simulink model "microgrid_healthy_load_profiling_with_Utility"  (Simulink 7.9)
settings: Solver=ode3  SolverMode=SingleTasking  StartTime=0.0  StopTime=12  FixedStep=1*10^(-4)  RelTol=1e-3
undefined symbols (not defined in the file): D1, Delta, Ts
libraries: powerlib x102, powerlib_extras x22
(part 1 of 2)
settings Model: Creator=SK  LastModifiedBy=SK
settings SolverCC: ZeroCrossAlgorithm=Adaptive  AlgebraicLoopSolver=LineSearch
settings OptimizationCC: SimCompilerOptimization=On  AccelVerboseBuild=on
settings SFSimCC: SFSimEnableDebug=off  SFSimEcho=off
settings RTWCC: RTWCompilerOptimization=On

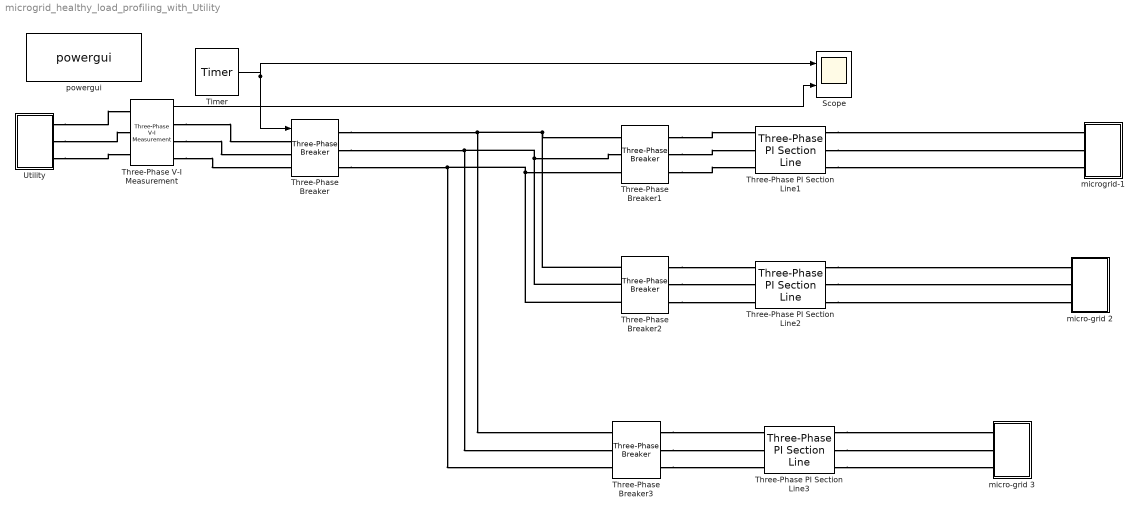
== system microgrid_healthy_load_profiling_with_Utility ==
  Scope : Scope  NumInputPorts=2
      settings: YMin=1~-55  YMax=1~55
  Three-Phase PI Section Line1 : powerlib/Elements/Three-Phase PI Section Line  LConnTagsString=a|b|c  RConnTagsString=A|B|C  Frequency=60  Resistances=[ 36.757 0.0]  Inductances="[ 0.126  0.0001]"  Capacitances=[0.00001 0.0001]  Length=2.06
  Three-Phase PI Section Line2 : powerlib/Elements/Three-Phase PI Section Line  LConnTagsString=a|b|c  RConnTagsString=A|B|C  Frequency=60  Resistances=[ 36.757 0.0]  Inductances="[ 0.126  0.0001]"  Capacitances=[0.00001 0.0001]  Length=2.06
  Three-Phase PI Section Line3 : powerlib/Elements/Three-Phase PI Section Line  LConnTagsString=a|b|c  RConnTagsString=A|B|C  Frequency=60  Resistances=[ 36.757 0.0]  Inductances="[ 0.126  0.0001]"  Capacitances=[0.00001 0.0001]  Length=2.06
  Three-Phase V-I Measurement : powerlib/Measurements/Three-Phase V-I Measurement  VoltageMeasurement=no  SetLabelV=off  LabelV=Vabc  Vpu=off  VpuLL=off  CurrentMeasurement=yes  SetLabelI=off  LabelI=Iabc  Ipu=off  Pbase=100e6  Vbase=500e3  OutputType=Magnitude  PhasorSimulation=off  PSBequivalent=0
  Three-Phase Breaker : powerlib/Elements/Three-Phase Breaker  InitialState=closed  SwitchA=on  SwitchB=on  SwitchC=on  SwitchTimes="[4/60  10/60]"  External=on  BreakerResistance=0.001  SnubberResistance=1e6  SnubberCapacitance=inf  Measurements=None
  Three-Phase Breaker1 : powerlib/Elements/Three-Phase Breaker  InitialState=open  SwitchA=off  SwitchB=off  SwitchC=off  SwitchTimes="[4/60  10/60]"  External=off  BreakerResistance=0.001  SnubberResistance=1e6  SnubberCapacitance=inf  Measurements=None
  Three-Phase Breaker2 : powerlib/Elements/Three-Phase Breaker  InitialState=open  SwitchA=off  SwitchB=off  SwitchC=off  SwitchTimes="[4/60  10/60]"  External=off  BreakerResistance=0.001  SnubberResistance=1e6  SnubberCapacitance=inf  Measurements=None
  Three-Phase Breaker3 : powerlib/Elements/Three-Phase Breaker  InitialState=open  SwitchA=off  SwitchB=off  SwitchC=off  SwitchTimes="[4/60  10/60]"  External=off  BreakerResistance=0.001  SnubberResistance=1e6  SnubberCapacitance=inf  Measurements=None
  Timer : powerlib_extras/Control  Blocks/Timer  t=[ 0 ]  e=[1]
  Utility : Subsystem
  micro-grid 2 : Subsystem
  micro-grid 3 : Subsystem
  microgrid-1 : Subsystem
  powergui : powerlib/powergui  Priority=1  SimulationMode=Discrete  SolverType=Tustin  SampleTime=Ts  frequency=60  SPID=on  DisableSnubberDevices=off  DisableRonSwitches=off  DisableVfSwitches=off  SwTol=0  Interpol=off  DisplayEquations=off  FunctionMessages=off  frequencyindice=60  Pbase=5e6  ErrMax=1e-4  Iterations=50  UnitsV=kV  UnitsW=MW  echomessages=off  HookPort=off  EnableUseOfTLC=off  x0status=blocks  RestoreLinks=warning  ResistiveCurrentMeasurement=off  Ylog=off  Xlog=on  ShowGrid=off  save=off  variable=ZData  structure=y  ZoomFFT=off  StartTime=0.0  cycles=1  DisplayStyle=1  fundamental=60  FreqAxis=off  MaxFrequency=1000  frequencyindicesteady=1  display=off  methode=off
  wires:
  Timer/1 -> Three-Phase Breaker/1, Scope/1
  Three-Phase V-I Measurement/1 -> Scope/2
  connections:
  Three-Phase V-I Measurement/RConn2 -- Three-Phase Breaker/LConn2
  Utility/RConn2 -- Three-Phase V-I Measurement/LConn2
  Three-Phase V-I Measurement/RConn1 -- Three-Phase Breaker/LConn1
  Three-Phase V-I Measurement/RConn3 -- Three-Phase Breaker/LConn3
  Utility/RConn1 -- Three-Phase V-I Measurement/LConn1
  Utility/RConn3 -- Three-Phase V-I Measurement/LConn3
  Three-Phase Breaker2/LConn1 -- Three-Phase Breaker/RConn1 -- Three-Phase Breaker3/LConn1 -- Three-Phase Breaker1/LConn1
  Three-Phase Breaker2/LConn2 -- Three-Phase Breaker/RConn2 -- Three-Phase Breaker3/LConn2 -- Three-Phase Breaker1/LConn2
  Three-Phase Breaker2/LConn3 -- Three-Phase Breaker/RConn3 -- Three-Phase Breaker3/LConn3 -- Three-Phase Breaker1/LConn3
  Three-Phase PI Section Line3/RConn1 -- micro-grid 3/LConn1
  Three-Phase PI Section Line3/RConn2 -- micro-grid 3/LConn2
  Three-Phase PI Section Line3/RConn3 -- micro-grid 3/LConn3
  Three-Phase PI Section Line1/RConn1 -- microgrid-1/LConn1
  Three-Phase PI Section Line1/RConn2 -- microgrid-1/LConn2
  Three-Phase PI Section Line1/RConn3 -- microgrid-1/LConn3
  Three-Phase PI Section Line2/RConn1 -- micro-grid 2/LConn1
  Three-Phase PI Section Line2/RConn2 -- micro-grid 2/LConn2
  Three-Phase PI Section Line2/RConn3 -- micro-grid 2/LConn3
  Three-Phase Breaker3/RConn1 -- Three-Phase PI Section Line3/LConn1
  Three-Phase Breaker3/RConn2 -- Three-Phase PI Section Line3/LConn2
  Three-Phase Breaker3/RConn3 -- Three-Phase PI Section Line3/LConn3
  Three-Phase Breaker2/RConn1 -- Three-Phase PI Section Line2/LConn1
  Three-Phase Breaker2/RConn2 -- Three-Phase PI Section Line2/LConn2
  Three-Phase Breaker2/RConn3 -- Three-Phase PI Section Line2/LConn3
  Three-Phase Breaker1/RConn1 -- Three-Phase PI Section Line1/LConn1
  Three-Phase Breaker1/RConn2 -- Three-Phase PI Section Line1/LConn2
  Three-Phase Breaker1/RConn3 -- Three-Phase PI Section Line1/LConn3

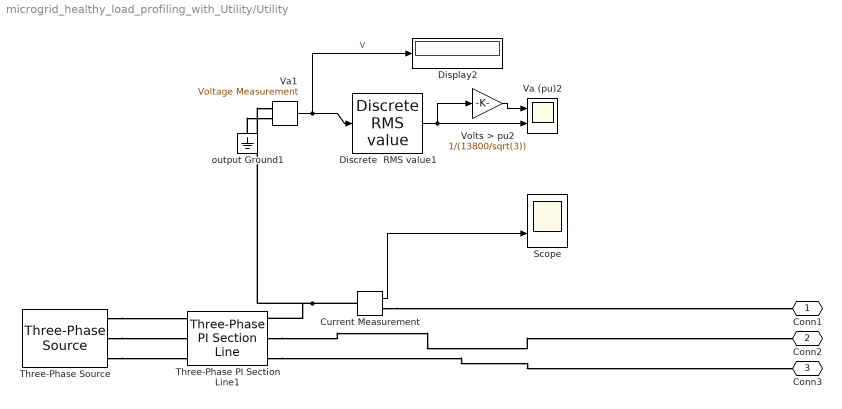
== system microgrid_healthy_load_profiling_with_Utility/Utility ==
  Current Measurement : powerlib/Measurements/Current Measurement  PhasorSimulation=off  OutputType=Complex  PSBequivalent=0
  Discrete  RMS value1 : powerlib_extras/Discrete Measurements/Discrete  RMS value  Freq=60  Mag_Init=0  Ts=Ts
  Display2 : Display
  Scope : Scope  NumInputPorts=2
      settings: YMin=-17500~-55  YMax=17500~55  SaveName=ScopeData2
  Three-Phase PI Section Line1 : powerlib/Elements/Three-Phase PI Section Line  LConnTagsString=a|b|c  RConnTagsString=A|B|C  Frequency=60  Resistances=[ 36.757 0.0]  Inductances="[ 0.126  0.0001]"  Capacitances=[0.00001 0.0001]  Length=2.06
  Three-Phase Source : powerlib/Electrical Sources/Three-Phase Source  Voltage=13.8e3  PhaseAngle=0  Frequency=60  InternalConnection=Yg  SpecifyImpedance=on  Resistance=0.8929  Inductance=16.58e-3  ShortCircuitLevel=1000e6  BaseVoltage=13.8e3  XRratio=22.2  BusType=swing  Pref=0  Qref=0  Qmin=-inf  Qmax=inf
  Va (pu)2 : Scope  NumInputPorts=2
      settings: TickLabels=on  TimeRange=3  YMin=1.35675~10809.8  YMax=1.35675~10809.8  SaveName=vf1
  Va1 : powerlib/Measurements/Voltage Measurement  Tag=PoWeRsYsTeMmEaSuReMeNt  PhasorSimulation=off  OutputType=Magnitude  PSBequivalent=0
  Volts > pu2 : Gain  Gain=1/(13800/sqrt(3))  SaturateOnIntegerOverflow=on  OutDataTypeStr=Inherit: Same as input  ParamDataTypeStr=Inherit: Same as input
  output Ground1 : powerlib/Elements/Ground  LConnTagsString=a
  Conn1 : PMIOPort  Port=1  Side=Right
  Conn2 : PMIOPort  Port=2  Side=Right
  Conn3 : PMIOPort  Port=3  Side=Right
  wires:
  Current Measurement/1 -> Scope/2
  Va1/1 -> Discrete  RMS value1/1, Display2/1  "V"
  Discrete  RMS value1/1 -> Va (pu)2/2, Volts > pu2/1
  Volts > pu2/1 -> Va (pu)2/1
  connections:
  Three-Phase Source/RConn1 -- Three-Phase PI Section Line1/LConn1
  Three-Phase Source/RConn2 -- Three-Phase PI Section Line1/LConn2
  Three-Phase Source/RConn3 -- Three-Phase PI Section Line1/LConn3
  Three-Phase PI Section Line1/RConn2 -- Conn2/RConn1
  Three-Phase PI Section Line1/RConn3 -- Conn3/RConn1
  Current Measurement/LConn1 -- Three-Phase PI Section Line1/RConn1 -- Va1/LConn1
  Current Measurement/RConn1 -- Conn1/RConn1
  output Ground1/LConn1 -- Va1/LConn2

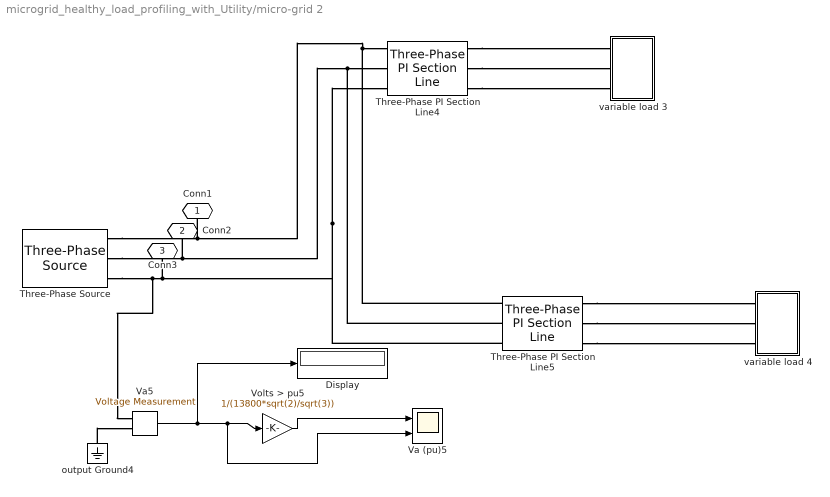
== system microgrid_healthy_load_profiling_with_Utility/micro-grid 2 ==
  Display : Display
  Three-Phase PI Section Line4 : powerlib/Elements/Three-Phase PI Section Line  LConnTagsString=a|b|c  RConnTagsString=A|B|C  Frequency=60  Resistances=[13.8 0.0]  Inductances="[ 0.046  0.0001]"  Capacitances=[0.00001 0.0001]  Length=0.148
  Three-Phase PI Section Line5 : powerlib/Elements/Three-Phase PI Section Line  LConnTagsString=a|b|c  RConnTagsString=A|B|C  Frequency=60  Resistances=[ 134.04 0.0]  Inductances="[ 0.046  0.0001]"  Capacitances=[0.00001 0.0001]  Length=0.104
  Three-Phase Source : powerlib/Electrical Sources/Three-Phase Source  Voltage=13.8e3  PhaseAngle=0  Frequency=60  InternalConnection=Yg  SpecifyImpedance=off  Resistance=0.198  Inductance=0.303  ShortCircuitLevel=1000e6  BaseVoltage=13.8e3  XRratio=22.2  BusType=PQ  Pref=4.5E6  Qref=1.5E6  Qmin=-inf  Qmax=inf
  Va (pu)5 : Scope  NumInputPorts=2
      settings: TickLabels=on  TimeRange=2  YMin=-1.1~-12500  YMax=1.1~12500  SaveName=vf
  Va5 : powerlib/Measurements/Voltage Measurement  Tag=PoWeRsYsTeMmEaSuReMeNt  PhasorSimulation=off  OutputType=Magnitude  PSBequivalent=0
  Volts > pu5 : Gain  Gain=1/(13800*sqrt(2)/sqrt(3))  SaturateOnIntegerOverflow=on  OutDataTypeStr=Inherit: Same as input  ParamDataTypeStr=Inherit: Same as input
  output Ground4 : powerlib/Elements/Ground  LConnTagsString=a
  variable load 3 : Subsystem
  variable load 4 : Subsystem
  Conn1 : PMIOPort  Port=1  Side=Left
  Conn2 : PMIOPort  Port=2  Side=Left
  Conn3 : PMIOPort  Port=3  Side=Left
  wires:
  Va5/1 -> Display/1, Va (pu)5/2, Volts > pu5/1
  Volts > pu5/1 -> Va (pu)5/1
  connections:
  output Ground4/LConn1 -- Va5/LConn2
  Va5/LConn1 -- Conn3/RConn1 -- Three-Phase PI Section Line4/LConn3 -- Three-Phase PI Section Line5/LConn3 -- Three-Phase Source/RConn3
  Three-Phase Source/RConn2 -- Conn2/RConn1 -- Three-Phase PI Section Line4/LConn2 -- Three-Phase PI Section Line5/LConn2
  Three-Phase Source/RConn1 -- Conn1/RConn1 -- Three-Phase PI Section Line4/LConn1 -- Three-Phase PI Section Line5/LConn1
  Three-Phase PI Section Line4/RConn1 -- variable load 3/LConn1
  Three-Phase PI Section Line4/RConn2 -- variable load 3/LConn2
  Three-Phase PI Section Line4/RConn3 -- variable load 3/LConn3
  Three-Phase PI Section Line5/RConn1 -- variable load 4/LConn1
  Three-Phase PI Section Line5/RConn2 -- variable load 4/LConn2
  Three-Phase PI Section Line5/RConn3 -- variable load 4/LConn3

== system microgrid_healthy_load_profiling_with_Utility/micro-grid 3 ==
  DG2 : Subsystem
  bus 3 : Subsystem
  Conn1 : PMIOPort  Port=1  Side=Left
  Conn2 : PMIOPort  Port=2  Side=Left
  Conn3 : PMIOPort  Port=3  Side=Left
  connections:
  Conn2/RConn1 -- DG2/LConn2 -- bus 3/LConn2
  Conn1/RConn1 -- DG2/LConn1 -- bus 3/LConn1
  Conn3/RConn1 -- DG2/LConn3 -- bus 3/LConn3

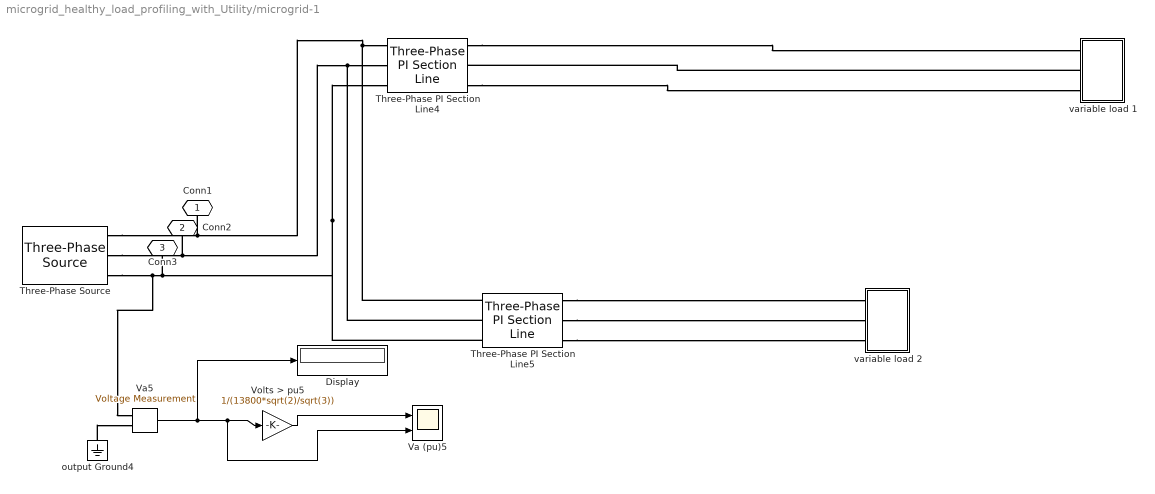
== system microgrid_healthy_load_profiling_with_Utility/microgrid-1 ==
  Display : Display
  Three-Phase PI Section Line4 : powerlib/Elements/Three-Phase PI Section Line  LConnTagsString=a|b|c  RConnTagsString=A|B|C  Frequency=60  Resistances=[13.8 0.0]  Inductances="[ 0.046  0.0001]"  Capacitances=[0.00001 0.0001]  Length=0.148
  Three-Phase PI Section Line5 : powerlib/Elements/Three-Phase PI Section Line  LConnTagsString=a|b|c  RConnTagsString=A|B|C  Frequency=60  Resistances=[ 134.04 0.0]  Inductances="[ 0.046  0.0001]"  Capacitances=[0.00001 0.0001]  Length=0.104
  Three-Phase Source : powerlib/Electrical Sources/Three-Phase Source  Voltage=13.8e3  PhaseAngle=0  Frequency=60  InternalConnection=Yg  SpecifyImpedance=off  Resistance=0.198  Inductance=0.303  ShortCircuitLevel=1000e6  BaseVoltage=13.8e3  XRratio=22.2  BusType=swing  Pref=4.5E6  Qref=1.5E6  Qmin=-inf  Qmax=inf
  Va (pu)5 : Scope  NumInputPorts=2
      settings: TickLabels=on  TimeRange=2  YMin=-0.054909~-618.696  YMax=-0.0496796~-559.772  SaveName=vf
  Va5 : powerlib/Measurements/Voltage Measurement  Tag=PoWeRsYsTeMmEaSuReMeNt  PhasorSimulation=off  OutputType=Magnitude  PSBequivalent=0
  Volts > pu5 : Gain  Gain=1/(13800*sqrt(2)/sqrt(3))  SaturateOnIntegerOverflow=on  OutDataTypeStr=Inherit: Same as input  ParamDataTypeStr=Inherit: Same as input
  output Ground4 : powerlib/Elements/Ground  LConnTagsString=a
  variable load 1 : Subsystem
  variable load 2 : Subsystem
  Conn1 : PMIOPort  Port=1  Side=Left
  Conn2 : PMIOPort  Port=2  Side=Left
  Conn3 : PMIOPort  Port=3  Side=Left
  wires:
  Va5/1 -> Volts > pu5/1, Va (pu)5/2, Display/1
  Volts > pu5/1 -> Va (pu)5/1
  connections:
  Conn1/RConn1 -- Three-Phase Source/RConn1 -- Three-Phase PI Section Line5/LConn1 -- Three-Phase PI Section Line4/LConn1
  Conn2/RConn1 -- Three-Phase Source/RConn2 -- Three-Phase PI Section Line5/LConn2 -- Three-Phase PI Section Line4/LConn2
  Conn3/RConn1 -- Three-Phase Source/RConn3 -- Va5/LConn1 -- Three-Phase PI Section Line5/LConn3 -- Three-Phase PI Section Line4/LConn3
  output Ground4/LConn1 -- Va5/LConn2
  variable load 1/LConn2 -- Three-Phase PI Section Line4/RConn2
  Three-Phase PI Section Line4/RConn3 -- variable load 1/LConn3
  Three-Phase PI Section Line4/RConn1 -- variable load 1/LConn1
  Three-Phase PI Section Line5/RConn1 -- variable load 2/LConn1
  Three-Phase PI Section Line5/RConn2 -- variable load 2/LConn2
  Three-Phase PI Section Line5/RConn3 -- variable load 2/LConn3

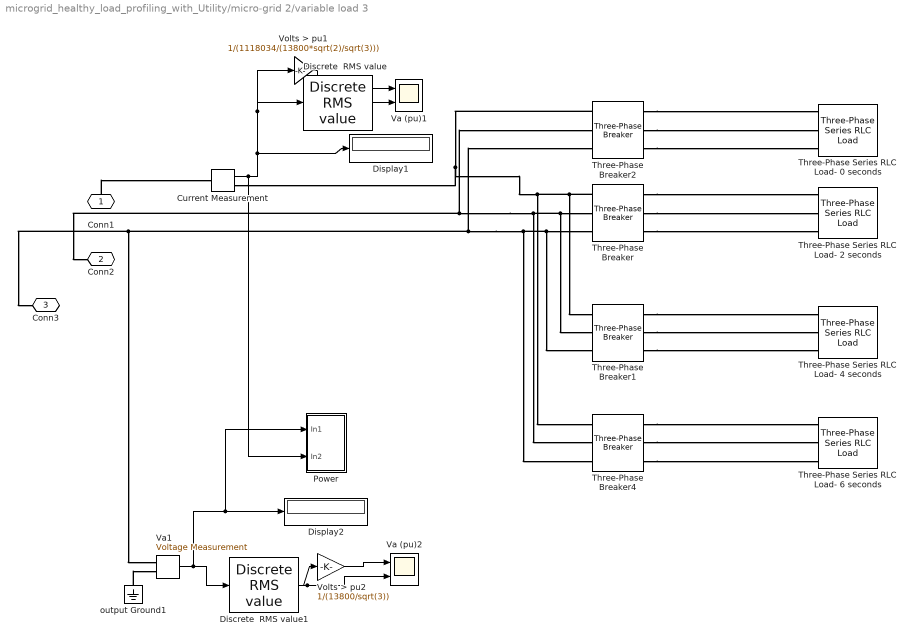
== system microgrid_healthy_load_profiling_with_Utility/micro-grid 2/variable load 3 ==
  Current Measurement : powerlib/Measurements/Current Measurement  PhasorSimulation=off  OutputType=Complex  PSBequivalent=0
  Discrete  RMS value : powerlib_extras/Discrete Measurements/Discrete  RMS value  Freq=60  Mag_Init=0  Ts=Ts
  Discrete  RMS value1 : powerlib_extras/Discrete Measurements/Discrete  RMS value  Freq=60  Mag_Init=0  Ts=Ts
  Display1 : Display
  Display2 : Display
  Power : Subsystem
  Three-Phase Series RLC Load- 0 seconds : powerlib/Elements/Three-Phase Series RLC Load  LConnTagsString=A|B|C  Configuration=Y (grounded)  NominalVoltage=13800  NominalFrequency=60  ActivePower=600e3  InductivePower=150e3  CapacitivePower=0  Measurements=None  LoadType=constant Z
  "Three-Phase Series RLC Load- 2 seconds " : powerlib/Elements/Three-Phase Series RLC Load  LConnTagsString=A|B|C  Configuration=Y (grounded)  NominalVoltage=13800  NominalFrequency=60  ActivePower=50e3  InductivePower=0  CapacitivePower=50e3  Measurements=None  LoadType=constant Z
  Three-Phase Series RLC Load- 4 seconds : powerlib/Elements/Three-Phase Series RLC Load  LConnTagsString=A|B|C  Configuration=Y (grounded)  NominalVoltage=13800  NominalFrequency=60  ActivePower=20e3  InductivePower=30e3  CapacitivePower=0  Measurements=None  LoadType=constant Z
  Three-Phase Series RLC Load- 6 seconds : powerlib/Elements/Three-Phase Series RLC Load  LConnTagsString=A|B|C  Configuration=Y (grounded)  NominalVoltage=13800  NominalFrequency=60  ActivePower=30e3  InductivePower=0  CapacitivePower=40e3  Measurements=None  LoadType=constant Z
  Three-Phase Breaker : powerlib/Elements/Three-Phase Breaker  InitialState=open  SwitchA=on  SwitchB=on  SwitchC=on  SwitchTimes="[180/60  360/60]"  External=off  BreakerResistance=0.001  SnubberResistance=1e6  SnubberCapacitance=inf  Measurements=None
  Three-Phase Breaker1 : powerlib/Elements/Three-Phase Breaker  InitialState=open  SwitchA=on  SwitchB=on  SwitchC=on  SwitchTimes="[360/60  540/60]"  External=off  BreakerResistance=0.001  SnubberResistance=1e6  SnubberCapacitance=inf  Measurements=None
  Three-Phase Breaker2 : powerlib/Elements/Three-Phase Breaker  InitialState=closed  SwitchA=off  SwitchB=off  SwitchC=off  SwitchTimes=[120/60 ]  External=off  BreakerResistance=0.001  SnubberResistance=1e6  SnubberCapacitance=inf  Measurements=None
  Three-Phase Breaker4 : powerlib/Elements/Three-Phase Breaker  InitialState=open  SwitchA=on  SwitchB=on  SwitchC=on  SwitchTimes=[540/60 ]  External=off  BreakerResistance=0.001  SnubberResistance=1e6  SnubberCapacitance=inf  Measurements=None
  Va (pu)1 : Scope  NumInputPorts=2
      settings: TickLabels=on  TimeRange=2  YMin=-0.8~-50  YMax=0.8~50  SaveName=vf6
  Va (pu)2 : Scope  NumInputPorts=2
      settings: TickLabels=on  TimeRange=2  YMin=-2~-12500  YMax=2~12500  SaveName=vf2
  Va1 : powerlib/Measurements/Voltage Measurement  Tag=PoWeRsYsTeMmEaSuReMeNt  PhasorSimulation=off  OutputType=Magnitude  PSBequivalent=0
  Volts > pu1 : Gain  Gain=1/(1118034/(13800*sqrt(2)/sqrt(3)))  SaturateOnIntegerOverflow=on  OutDataTypeStr=Inherit: Same as input  ParamDataTypeStr=Inherit: Same as input
  Volts > pu2 : Gain  Gain=1/(13800/sqrt(3))  SaturateOnIntegerOverflow=on  OutDataTypeStr=Inherit: Same as input  ParamDataTypeStr=Inherit: Same as input
  output Ground1 : powerlib/Elements/Ground  LConnTagsString=a
  Conn1 : PMIOPort  Port=1  Side=Left
  Conn2 : PMIOPort  Port=2  Side=Left
  Conn3 : PMIOPort  Port=3  Side=Left
  wires:
  Current Measurement/1 -> Display1/1, Volts > pu1/1, Discrete  RMS value/1, Power/2(In2)
  Volts > pu1/1 -> Va (pu)1/1
  Va1/1 -> Display2/1, Power/1(In1), Discrete  RMS value1/1
  Discrete  RMS value/1 -> Va (pu)1/2
  Discrete  RMS value1/1 -> Va (pu)2/2, Volts > pu2/1
  Volts > pu2/1 -> Va (pu)2/1
  connections:
  Conn1/RConn1 -- Current Measurement/LConn1
  output Ground1/LConn1 -- Va1/LConn2
  Three-Phase Breaker2/RConn3 -- Three-Phase Series RLC Load- 0 seconds/LConn3
  Three-Phase Breaker2/RConn2 -- Three-Phase Series RLC Load- 0 seconds/LConn2
  Three-Phase Breaker2/RConn1 -- Three-Phase Series RLC Load- 0 seconds/LConn1
  Va1/LConn1 -- Conn3/RConn1 -- Three-Phase Breaker2/LConn3 -- Three-Phase Breaker4/LConn3 -- Three-Phase Breaker1/LConn3 -- Three-Phase Breaker/LConn3
  Three-Phase Breaker2/LConn2 -- Conn2/RConn1 -- Three-Phase Breaker4/LConn2 -- Three-Phase Breaker1/LConn2 -- Three-Phase Breaker/LConn2
  Current Measurement/RConn1 -- Three-Phase Breaker2/LConn1 -- Three-Phase Breaker4/LConn1 -- Three-Phase Breaker1/LConn1 -- Three-Phase Breaker/LConn1
  Three-Phase Breaker4/RConn3 -- Three-Phase Series RLC Load- 6 seconds/LConn3
  Three-Phase Breaker4/RConn2 -- Three-Phase Series RLC Load- 6 seconds/LConn2
  Three-Phase Breaker4/RConn1 -- Three-Phase Series RLC Load- 6 seconds/LConn1
  Three-Phase Breaker1/RConn3 -- Three-Phase Series RLC Load- 4 seconds/LConn3
  Three-Phase Breaker1/RConn2 -- Three-Phase Series RLC Load- 4 seconds/LConn2
  Three-Phase Breaker1/RConn1 -- Three-Phase Series RLC Load- 4 seconds/LConn1
  Three-Phase Breaker/RConn3 -- "Three-Phase Series RLC Load- 2 seconds "/LConn3
  Three-Phase Breaker/RConn2 -- "Three-Phase Series RLC Load- 2 seconds "/LConn2
  Three-Phase Breaker/RConn1 -- "Three-Phase Series RLC Load- 2 seconds "/LConn1

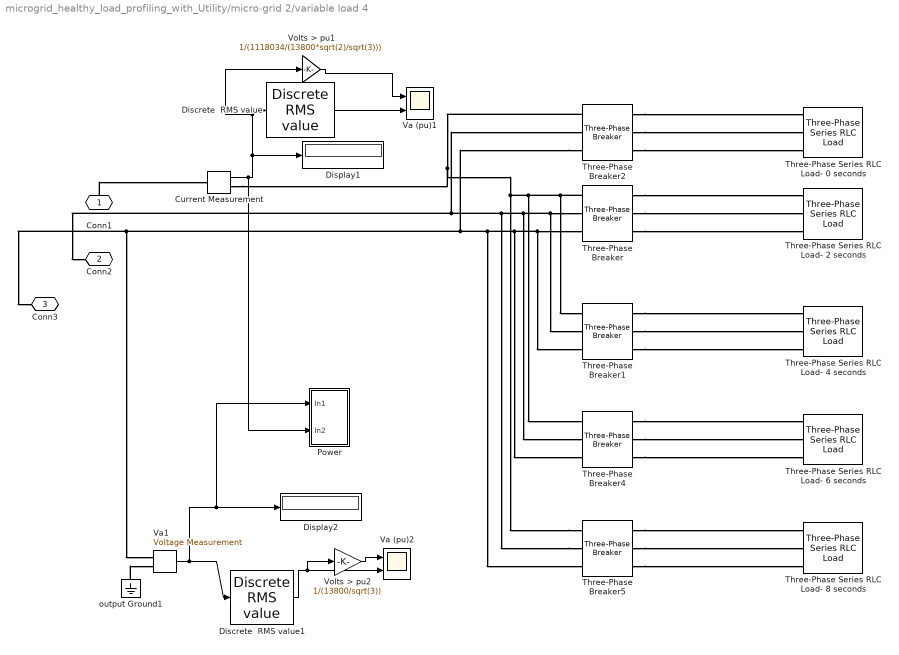
== system microgrid_healthy_load_profiling_with_Utility/micro-grid 2/variable load 4 ==
  Current Measurement : powerlib/Measurements/Current Measurement  PhasorSimulation=off  OutputType=Complex  PSBequivalent=0
  Discrete  RMS value : powerlib_extras/Discrete Measurements/Discrete  RMS value  Freq=60  Mag_Init=0  Ts=Ts
  Discrete  RMS value1 : powerlib_extras/Discrete Measurements/Discrete  RMS value  Freq=60  Mag_Init=0  Ts=Ts
  Display1 : Display
  Display2 : Display
  Power : Subsystem
  Three-Phase Series RLC Load- 0 seconds : powerlib/Elements/Three-Phase Series RLC Load  LConnTagsString=A|B|C  Configuration=Y (grounded)  NominalVoltage=13800  NominalFrequency=60  ActivePower=650e3  InductivePower=150e3  CapacitivePower=0  Measurements=None  LoadType=constant Z
  "Three-Phase Series RLC Load- 2 seconds " : powerlib/Elements/Three-Phase Series RLC Load  LConnTagsString=A|B|C  Configuration=Y (grounded)  NominalVoltage=13800  NominalFrequency=60  ActivePower=650e3  InductivePower=100e3  CapacitivePower=0  Measurements=None  LoadType=constant Z
  Three-Phase Series RLC Load- 4 seconds : powerlib/Elements/Three-Phase Series RLC Load  LConnTagsString=A|B|C  Configuration=Y (grounded)  NominalVoltage=13800  NominalFrequency=60  ActivePower=600e3  InductivePower=150e3  CapacitivePower=0  Measurements=None  LoadType=constant Z
  Three-Phase Series RLC Load- 6 seconds : powerlib/Elements/Three-Phase Series RLC Load  LConnTagsString=A|B|C  Configuration=Y (grounded)  NominalVoltage=13800  NominalFrequency=60  ActivePower=650e3  InductivePower=100e3  CapacitivePower=0  Measurements=None  LoadType=constant Z
  Three-Phase Series RLC Load- 8 seconds : powerlib/Elements/Three-Phase Series RLC Load  LConnTagsString=A|B|C  Configuration=Y (grounded)  NominalVoltage=13800  NominalFrequency=60  ActivePower=0.5e6  InductivePower=0.04e6  CapacitivePower=0  Measurements=None  LoadType=constant Z
  Three-Phase Breaker : powerlib/Elements/Three-Phase Breaker  InitialState=open  SwitchA=on  SwitchB=on  SwitchC=on  SwitchTimes="[120/60  240/60]"  External=off  BreakerResistance=0.001  SnubberResistance=1e6  SnubberCapacitance=inf  Measurements=None
  Three-Phase Breaker1 : powerlib/Elements/Three-Phase Breaker  InitialState=open  SwitchA=on  SwitchB=on  SwitchC=on  SwitchTimes="[240/60  360/60]"  External=off  BreakerResistance=0.001  SnubberResistance=1e6  SnubberCapacitance=inf  Measurements=None
  Three-Phase Breaker2 : powerlib/Elements/Three-Phase Breaker  InitialState=closed  SwitchA=off  SwitchB=off  SwitchC=off  SwitchTimes=[120/60 ]  External=off  BreakerResistance=0.001  SnubberResistance=1e6  SnubberCapacitance=inf  Measurements=None
  Three-Phase Breaker4 : powerlib/Elements/Three-Phase Breaker  InitialState=open  SwitchA=on  SwitchB=on  SwitchC=on  SwitchTimes="[360/60  480/60]"  External=off  BreakerResistance=0.001  SnubberResistance=1e6  SnubberCapacitance=inf  Measurements=None
  Three-Phase Breaker5 : powerlib/Elements/Three-Phase Breaker  InitialState=open  SwitchA=on  SwitchB=on  SwitchC=on  SwitchTimes=[480/60 ]  External=off  BreakerResistance=0.001  SnubberResistance=1e6  SnubberCapacitance=inf  Measurements=None
  Va (pu)1 : Scope  NumInputPorts=2
      settings: TickLabels=on  TimeRange=2  YMin=-0.8~-50  YMax=0.8~50  SaveName=vf6
  Va (pu)2 : Scope  NumInputPorts=2
      settings: TickLabels=on  TimeRange=2  YMin=-2~-12500  YMax=2~12500  SaveName=vf2
  Va1 : powerlib/Measurements/Voltage Measurement  Tag=PoWeRsYsTeMmEaSuReMeNt  PhasorSimulation=off  OutputType=Magnitude  PSBequivalent=0
  Volts > pu1 : Gain  Gain=1/(1118034/(13800*sqrt(2)/sqrt(3)))  SaturateOnIntegerOverflow=on  OutDataTypeStr=Inherit: Same as input  ParamDataTypeStr=Inherit: Same as input
  Volts > pu2 : Gain  Gain=1/(13800/sqrt(3))  SaturateOnIntegerOverflow=on  OutDataTypeStr=Inherit: Same as input  ParamDataTypeStr=Inherit: Same as input
  output Ground1 : powerlib/Elements/Ground  LConnTagsString=a
  Conn1 : PMIOPort  Port=1  Side=Left
  Conn2 : PMIOPort  Port=2  Side=Left
  Conn3 : PMIOPort  Port=3  Side=Left
  wires:
  Va1/1 -> Display2/1, Power/1(In1), Discrete  RMS value1/1
  Volts > pu1/1 -> Va (pu)1/1
  Current Measurement/1 -> Volts > pu1/1, Discrete  RMS value/1, Display1/1, Power/2(In2)
  Discrete  RMS value/1 -> Va (pu)1/2
  Discrete  RMS value1/1 -> Va (pu)2/2, Volts > pu2/1
  Volts > pu2/1 -> Va (pu)2/1
  connections:
  Three-Phase Breaker/RConn1 -- "Three-Phase Series RLC Load- 2 seconds "/LConn1
  Three-Phase Breaker/RConn2 -- "Three-Phase Series RLC Load- 2 seconds "/LConn2
  Three-Phase Breaker/RConn3 -- "Three-Phase Series RLC Load- 2 seconds "/LConn3
  Three-Phase Breaker1/RConn1 -- Three-Phase Series RLC Load- 4 seconds/LConn1
  Three-Phase Breaker1/RConn2 -- Three-Phase Series RLC Load- 4 seconds/LConn2
  Three-Phase Breaker1/RConn3 -- Three-Phase Series RLC Load- 4 seconds/LConn3
  Three-Phase Breaker4/RConn1 -- Three-Phase Series RLC Load- 6 seconds/LConn1
  Three-Phase Breaker4/RConn2 -- Three-Phase Series RLC Load- 6 seconds/LConn2
  Three-Phase Breaker4/RConn3 -- Three-Phase Series RLC Load- 6 seconds/LConn3
  Three-Phase Breaker5/RConn1 -- Three-Phase Series RLC Load- 8 seconds/LConn1
  Three-Phase Breaker5/RConn2 -- Three-Phase Series RLC Load- 8 seconds/LConn2
  Three-Phase Breaker5/RConn3 -- Three-Phase Series RLC Load- 8 seconds/LConn3
  Three-Phase Breaker5/LConn1 -- Three-Phase Breaker2/LConn1 -- Current Measurement/RConn1 -- Three-Phase Breaker/LConn1 -- Three-Phase Breaker1/LConn1 -- Three-Phase Breaker4/LConn1
  Three-Phase Breaker5/LConn2 -- Conn2/RConn1 -- Three-Phase Breaker2/LConn2 -- Three-Phase Breaker/LConn2 -- Three-Phase Breaker1/LConn2 -- Three-Phase Breaker4/LConn2
  Three-Phase Breaker2/LConn3 -- Conn3/RConn1 -- Va1/LConn1 -- Three-Phase Breaker/LConn3 -- Three-Phase Breaker1/LConn3 -- Three-Phase Breaker4/LConn3 -- Three-Phase Breaker5/LConn3
  Three-Phase Breaker2/RConn1 -- Three-Phase Series RLC Load- 0 seconds/LConn1
  Three-Phase Breaker2/RConn2 -- Three-Phase Series RLC Load- 0 seconds/LConn2
  Three-Phase Breaker2/RConn3 -- Three-Phase Series RLC Load- 0 seconds/LConn3
  output Ground1/LConn1 -- Va1/LConn2
  Conn1/RConn1 -- Current Measurement/LConn1

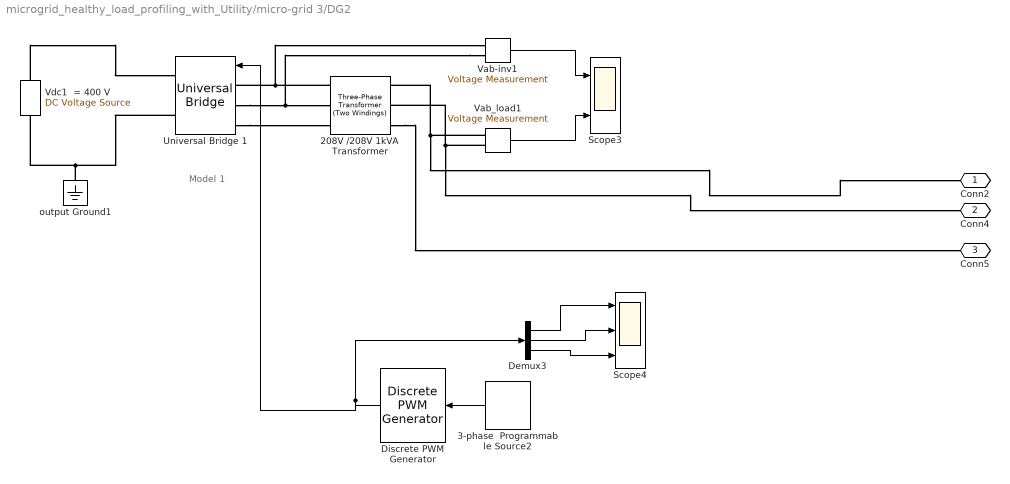
== system microgrid_healthy_load_profiling_with_Utility/micro-grid 3/DG2 ==
  note: Model 1
  208V /208V 1kVA Transformer : powerlib/Elements/Three-Phase Transformer (Two Windings)  Winding1Connection=Delta (D1)  UNITS=pu  NominalPower=[ 2.5e6 , 60 ]  Winding1=[ 480 ,0.01 , 0.15 ]  Winding2Connection=Yg  Winding2=[ 13800 , 0.01 , 0.15 ]  SetSaturation=off  Rm=200  Lm=200  Saturation="[ 0,0  ;  0.005,1.2  ;  1.0,1.4 ]"  Hysteresis=off  DataFile='hysteresis'  SetInitialFlux=off  InitialFluxes=[ 0.8 , -0.8 , 0.7 ]  Measurements=None  MoreParameters=off  BreakLoop=off  DataType=off  TransfoNumber=0
  3-phase  Programmable Source2 : powerlib_extras/Control  Blocks/3-phase  Programmable Source  Par_Vps=[480 0 60]  VariationEntity=None  VariationType=Ramp  VariationStep=-0.5  VariationRate=10  VariationMag=0.3  VariationFreq=2  Par_Timing_Variation=[0.2 1.2]  SinglePhase=off  Yampli=[1 0.8 1.2 1.0]  Xtime=[0 0.1 0.15 0.2]  HarmonicGeneration=off  Par_HarmoA="[3 5   -25 0]"  Par_HarmoB="[5  8   35  2]"  Par_Timing_Harmo="[ 0.05  99]"
  Demux3 : Demux  Outputs=3
  Discrete PWM Generator : powerlib_extras/Discrete  Control Blocks/Discrete PWM Generator  GeneratorMode="3-arm  bridge (6 pulses)"  Fc=1260  Ts=Ts  Internal=off  mIndex=0.4  Freq=60  Phase=0
  Scope3 : Scope  NumInputPorts=2
      settings: TickLabels=on  TimeRange=0.1  YMin=-400~-17500  YMax=400~17500  SaveName=Filter_out1
  Scope4 : Scope  NumInputPorts=3
      settings: TickLabels=on  TimeRange=0.1  YMin=-125~-125~-125  YMax=125~125~125  SaveName=Filter_out
  Universal Bridge 1 : powerlib/Power Electronics/Universal Bridge  Arms=3  SnubberResistance=10000  SnubberCapacitance=inf  Device=IGBT / Diodes  Ron=1e-4  Lon=0  ForwardVoltages="[  1  1  ]"  ForwardVoltage=.8  GTOparameters=[ 10e-6 , 20e-6 ]  IGBTparameters=[ 1e-6 , 2e-6 ]  Measurements=None  Measurements_2=None  converterType=Rectifier
      settings: AttributesFormatString=Device: %<Device>
  Vab-inv1 : powerlib/Measurements/Voltage Measurement  Tag=PoWeRsYsTeMmEaSuReMeNt  PhasorSimulation=off  OutputType=Magnitude  PSBequivalent=0
  Vab_load1 : powerlib/Measurements/Voltage Measurement  Tag=PoWeRsYsTeMmEaSuReMeNt  PhasorSimulation=off  OutputType=Magnitude  PSBequivalent=0
  Vdc1  = 400 V : powerlib/Electrical Sources/DC Voltage Source  Description=source block  Amplitude=400  Measurements=None
      settings: AttributesFormatString=\n
  output Ground1 : powerlib/Elements/Ground  LConnTagsString=a
  Conn2 : PMIOPort  Port=1  Side=Left
  Conn4 : PMIOPort  Port=2  Side=Left
  Conn5 : PMIOPort  Port=3  Side=Left
  wires:
  Vab-inv1/1 -> Scope3/1
  Vab_load1/1 -> Scope3/2
  Demux3/1 -> Scope4/1
  Demux3/2 -> Scope4/2
  Demux3/3 -> Scope4/3
  3-phase  Programmable Source2/1 -> Discrete PWM Generator/1
  Discrete PWM Generator/1 -> Demux3/1, Universal Bridge 1/1
  connections:
  Vab-inv1/LConn2 -- 208V /208V 1kVA Transformer/LConn2 -- Universal Bridge 1/LConn2
  208V /208V 1kVA Transformer/RConn1 -- Conn2/RConn1 -- Vab_load1/LConn1
  208V /208V 1kVA Transformer/RConn2 -- Conn4/RConn1 -- Vab_load1/LConn2
  Vdc1  = 400 V/LConn1 -- Universal Bridge 1/RConn2 -- output Ground1/LConn1
  Universal Bridge 1/LConn1 -- Vab-inv1/LConn1 -- 208V /208V 1kVA Transformer/LConn1
  Vdc1  = 400 V/RConn1 -- Universal Bridge 1/RConn1
  Universal Bridge 1/LConn3 -- 208V /208V 1kVA Transformer/LConn3
  208V /208V 1kVA Transformer/RConn3 -- Conn5/RConn1

== system microgrid_healthy_load_profiling_with_Utility/micro-grid 3/bus 3 ==
  Three-Phase PI Section Line1 : powerlib/Elements/Three-Phase PI Section Line  LConnTagsString=a|b|c  RConnTagsString=A|B|C  Frequency=60  Resistances=[13.8 0.0]  Inductances="[ 0.046  0.0001]"  Capacitances=[0.00001 0.0001]  Length=0.148
  Three-Phase PI Section Line2 : powerlib/Elements/Three-Phase PI Section Line  LConnTagsString=a|b|c  RConnTagsString=A|B|C  Frequency=60  Resistances=[ 134.04 0.0]  Inductances="[ 0.046  0.0001]"  Capacitances=[0.00001 0.0001]  Length=0.104
  variable load 5 : Subsystem
  variable load 6 : Subsystem
  Conn1 : PMIOPort  Port=1  Side=Left
  Conn2 : PMIOPort  Port=2  Side=Left
  Conn3 : PMIOPort  Port=3  Side=Left
  connections:
  Three-Phase PI Section Line2/LConn1 -- Conn1/RConn1 -- Three-Phase PI Section Line1/LConn1
  Three-Phase PI Section Line2/LConn2 -- Conn2/RConn1 -- Three-Phase PI Section Line1/LConn2
  Three-Phase PI Section Line2/LConn3 -- Conn3/RConn1 -- Three-Phase PI Section Line1/LConn3
  Three-Phase PI Section Line1/RConn1 -- variable load 5/LConn1
  Three-Phase PI Section Line1/RConn2 -- variable load 5/LConn2
  Three-Phase PI Section Line1/RConn3 -- variable load 5/LConn3
  Three-Phase PI Section Line2/RConn1 -- variable load 6/LConn1
  Three-Phase PI Section Line2/RConn2 -- variable load 6/LConn2
  Three-Phase PI Section Line2/RConn3 -- variable load 6/LConn3

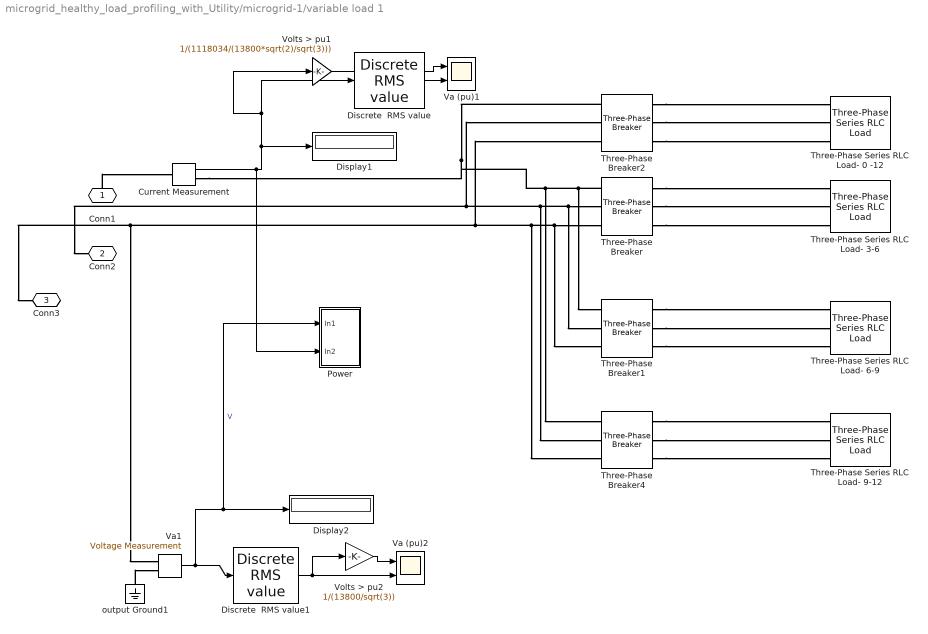
== system microgrid_healthy_load_profiling_with_Utility/microgrid-1/variable load 1 ==
  Current Measurement : powerlib/Measurements/Current Measurement  PhasorSimulation=off  OutputType=Complex  PSBequivalent=0
  Discrete  RMS value : powerlib_extras/Discrete Measurements/Discrete  RMS value  Freq=60  Mag_Init=0  Ts=Ts
  Discrete  RMS value1 : powerlib_extras/Discrete Measurements/Discrete  RMS value  Freq=60  Mag_Init=0  Ts=Ts
  Display1 : Display
  Display2 : Display
  Power : Subsystem
  Three-Phase Series RLC Load- 0 -12 : powerlib/Elements/Three-Phase Series RLC Load  LConnTagsString=A|B|C  Configuration=Y (grounded)  NominalVoltage=13800  NominalFrequency=60  ActivePower=550e3  InductivePower=175e3  CapacitivePower=0  Measurements=None  LoadType=constant Z
  Three-Phase Series RLC Load- 3-6 : powerlib/Elements/Three-Phase Series RLC Load  LConnTagsString=A|B|C  Configuration=Y (grounded)  NominalVoltage=13800  NominalFrequency=60  ActivePower=150e3  InductivePower=75e3  CapacitivePower=0  Measurements=None  LoadType=constant Z
  Three-Phase Series RLC Load- 6-9 : powerlib/Elements/Three-Phase Series RLC Load  LConnTagsString=A|B|C  Configuration=Y (grounded)  NominalVoltage=13800  NominalFrequency=60  ActivePower=250e3  InductivePower=0  CapacitivePower=50e3  Measurements=None  LoadType=constant Z
  Three-Phase Series RLC Load- 9-12 : powerlib/Elements/Three-Phase Series RLC Load  LConnTagsString=A|B|C  Configuration=Y (grounded)  NominalVoltage=13800  NominalFrequency=60  ActivePower=50e3  InductivePower=10e3  CapacitivePower=0  Measurements=None  LoadType=constant Z
  Three-Phase Breaker : powerlib/Elements/Three-Phase Breaker  InitialState=open  SwitchA=on  SwitchB=on  SwitchC=on  SwitchTimes="[180/60  360/60]"  External=off  BreakerResistance=0.001  SnubberResistance=1e6  SnubberCapacitance=inf  Measurements=None
  Three-Phase Breaker1 : powerlib/Elements/Three-Phase Breaker  InitialState=open  SwitchA=on  SwitchB=on  SwitchC=on  SwitchTimes="[360/60  540/60]"  External=off  BreakerResistance=0.001  SnubberResistance=1e6  SnubberCapacitance=inf  Measurements=None
  Three-Phase Breaker2 : powerlib/Elements/Three-Phase Breaker  InitialState=closed  SwitchA=off  SwitchB=off  SwitchC=off  SwitchTimes=[0 ]  External=off  BreakerResistance=0.001  SnubberResistance=1e6  SnubberCapacitance=inf  Measurements=None
  Three-Phase Breaker4 : powerlib/Elements/Three-Phase Breaker  InitialState=open  SwitchA=on  SwitchB=on  SwitchC=on  SwitchTimes=[540/60 ]  External=off  BreakerResistance=0.001  SnubberResistance=1e6  SnubberCapacitance=inf  Measurements=None
  Va (pu)1 : Scope  NumInputPorts=2
      settings: TickLabels=on  TimeRange=2  YMin=-0.55~36.7923  YMax=0.55~36.7923  SaveName=vf6
  Va (pu)2 : Scope  NumInputPorts=2
      settings: TickLabels=on  TimeRange=3  YMin=1.35675~10809.8  YMax=1.35675~10809.8  SaveName=vf2
  Va1 : powerlib/Measurements/Voltage Measurement  Tag=PoWeRsYsTeMmEaSuReMeNt  PhasorSimulation=off  OutputType=Magnitude  PSBequivalent=0
  Volts > pu1 : Gain  Gain=1/(1118034/(13800*sqrt(2)/sqrt(3)))  SaturateOnIntegerOverflow=on  OutDataTypeStr=Inherit: Same as input  ParamDataTypeStr=Inherit: Same as input
  Volts > pu2 : Gain  Gain=1/(13800/sqrt(3))  SaturateOnIntegerOverflow=on  OutDataTypeStr=Inherit: Same as input  ParamDataTypeStr=Inherit: Same as input
  output Ground1 : powerlib/Elements/Ground  LConnTagsString=a
  Conn1 : PMIOPort  Port=1  Side=Left
  Conn2 : PMIOPort  Port=2  Side=Left
  Conn3 : PMIOPort  Port=3  Side=Left
  wires:
  Va1/1 -> Display2/1, Power/1(In1), Discrete  RMS value1/1  "V"
  Volts > pu1/1 -> Va (pu)1/1
  Current Measurement/1 -> Display1/1, Volts > pu1/1, Discrete  RMS value/1, Power/2(In2)
  Discrete  RMS value/1 -> Va (pu)1/2
  Discrete  RMS value1/1 -> Va (pu)2/2, Volts > pu2/1
  Volts > pu2/1 -> Va (pu)2/1
  connections:
  Three-Phase Breaker/RConn1 -- Three-Phase Series RLC Load- 3-6/LConn1
  Three-Phase Breaker/RConn2 -- Three-Phase Series RLC Load- 3-6/LConn2
  Three-Phase Breaker/RConn3 -- Three-Phase Series RLC Load- 3-6/LConn3
  Three-Phase Breaker1/RConn1 -- Three-Phase Series RLC Load- 6-9/LConn1
  Three-Phase Breaker1/RConn2 -- Three-Phase Series RLC Load- 6-9/LConn2
  Three-Phase Breaker1/RConn3 -- Three-Phase Series RLC Load- 6-9/LConn3
  Three-Phase Breaker4/RConn1 -- Three-Phase Series RLC Load- 9-12/LConn1
  Three-Phase Breaker4/RConn2 -- Three-Phase Series RLC Load- 9-12/LConn2
  Three-Phase Breaker4/RConn3 -- Three-Phase Series RLC Load- 9-12/LConn3
  Three-Phase Breaker/LConn1 -- Three-Phase Breaker1/LConn1 -- Three-Phase Breaker4/LConn1 -- Three-Phase Breaker2/LConn1 -- Current Measurement/RConn1
  Three-Phase Breaker/LConn2 -- Three-Phase Breaker1/LConn2 -- Three-Phase Breaker4/LConn2 -- Conn2/RConn1 -- Three-Phase Breaker2/LConn2
  Three-Phase Breaker/LConn3 -- Three-Phase Breaker1/LConn3 -- Three-Phase Breaker4/LConn3 -- Conn3/RConn1 -- Va1/LConn1 -- Three-Phase Breaker2/LConn3
  Three-Phase Breaker2/RConn1 -- Three-Phase Series RLC Load- 0 -12/LConn1
  Three-Phase Breaker2/RConn2 -- Three-Phase Series RLC Load- 0 -12/LConn2
  Three-Phase Breaker2/RConn3 -- Three-Phase Series RLC Load- 0 -12/LConn3
  output Ground1/LConn1 -- Va1/LConn2
  Conn1/RConn1 -- Current Measurement/LConn1

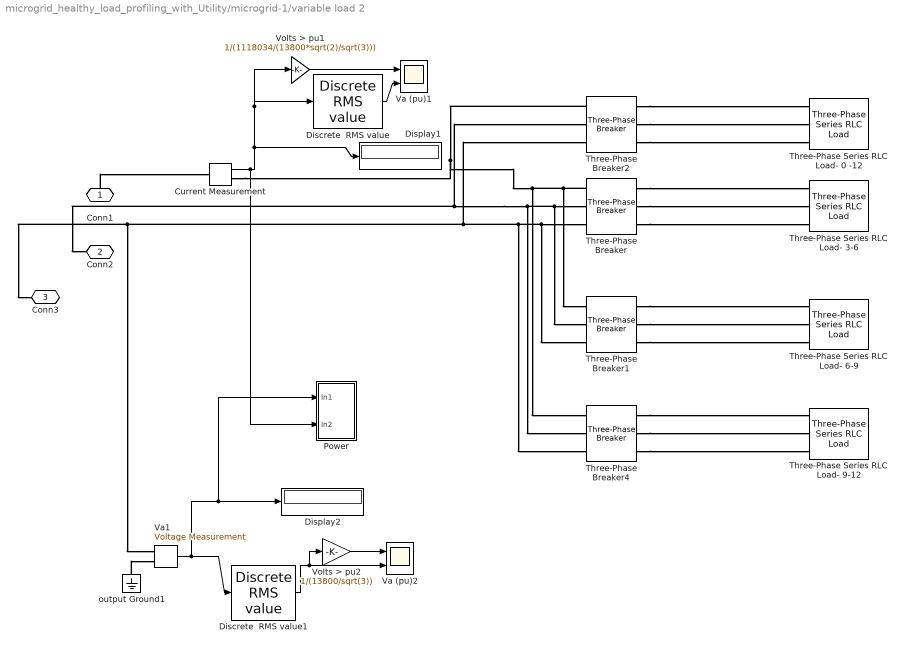
== system microgrid_healthy_load_profiling_with_Utility/microgrid-1/variable load 2 ==
  Current Measurement : powerlib/Measurements/Current Measurement  PhasorSimulation=off  OutputType=Complex  PSBequivalent=0
  Discrete  RMS value : powerlib_extras/Discrete Measurements/Discrete  RMS value  Freq=60  Mag_Init=0  Ts=Ts
  Discrete  RMS value1 : powerlib_extras/Discrete Measurements/Discrete  RMS value  Freq=60  Mag_Init=0  Ts=Ts
  Display1 : Display
  Display2 : Display
  Power : Subsystem
  Three-Phase Series RLC Load- 0 -12 : powerlib/Elements/Three-Phase Series RLC Load  LConnTagsString=A|B|C  Configuration=Y (grounded)  NominalVoltage=13800  NominalFrequency=60  ActivePower=650e3  InductivePower=100e3  CapacitivePower=0  Measurements=None  LoadType=constant Z
  Three-Phase Series RLC Load- 3-6 : powerlib/Elements/Three-Phase Series RLC Load  LConnTagsString=A|B|C  Configuration=Y (grounded)  NominalVoltage=13800  NominalFrequency=60  ActivePower=150e3  InductivePower=75e3  CapacitivePower=0  Measurements=None  LoadType=constant Z
  Three-Phase Series RLC Load- 6-9 : powerlib/Elements/Three-Phase Series RLC Load  LConnTagsString=A|B|C  Configuration=Y (grounded)  NominalVoltage=13800  NominalFrequency=60  ActivePower=300e3  InductivePower=90e3  CapacitivePower=0  Measurements=None  LoadType=constant Z
  Three-Phase Series RLC Load- 9-12 : powerlib/Elements/Three-Phase Series RLC Load  LConnTagsString=A|B|C  Configuration=Y (grounded)  NominalVoltage=13800  NominalFrequency=60  ActivePower=150e3  InductivePower=50e3  CapacitivePower=0  Measurements=None  LoadType=constant Z
  Three-Phase Breaker : powerlib/Elements/Three-Phase Breaker  InitialState=open  SwitchA=on  SwitchB=on  SwitchC=on  SwitchTimes="[180/60  360/60]"  External=off  BreakerResistance=0.001  SnubberResistance=1e6  SnubberCapacitance=inf  Measurements=None
  Three-Phase Breaker1 : powerlib/Elements/Three-Phase Breaker  InitialState=open  SwitchA=on  SwitchB=on  SwitchC=on  SwitchTimes="[360/60  540/60]"  External=off  BreakerResistance=0.001  SnubberResistance=1e6  SnubberCapacitance=inf  Measurements=None
  Three-Phase Breaker2 : powerlib/Elements/Three-Phase Breaker  InitialState=closed  SwitchA=off  SwitchB=off  SwitchC=off  SwitchTimes=[120/60 ]  External=off  BreakerResistance=0.001  SnubberResistance=1e6  SnubberCapacitance=inf  Measurements=None
  Three-Phase Breaker4 : powerlib/Elements/Three-Phase Breaker  InitialState=open  SwitchA=on  SwitchB=on  SwitchC=on  SwitchTimes=[540/60 ]  External=off  BreakerResistance=0.001  SnubberResistance=1e6  SnubberCapacitance=inf  Measurements=None
  Va (pu)1 : Scope  NumInputPorts=2
      settings: TickLabels=on  TimeRange=2  YMin=-0.8~-50  YMax=0.8~50  SaveName=vf6
  Va (pu)2 : Scope  NumInputPorts=2
      settings: TickLabels=on  TimeRange=2  YMin=1.18769~9462.9  YMax=1.18777~9463.5  SaveName=vf2
  Va1 : powerlib/Measurements/Voltage Measurement  Tag=PoWeRsYsTeMmEaSuReMeNt  PhasorSimulation=off  OutputType=Magnitude  PSBequivalent=0
  Volts > pu1 : Gain  Gain=1/(1118034/(13800*sqrt(2)/sqrt(3)))  SaturateOnIntegerOverflow=on  OutDataTypeStr=Inherit: Same as input  ParamDataTypeStr=Inherit: Same as input
  Volts > pu2 : Gain  Gain=1/(13800/sqrt(3))  SaturateOnIntegerOverflow=on  OutDataTypeStr=Inherit: Same as input  ParamDataTypeStr=Inherit: Same as input
  output Ground1 : powerlib/Elements/Ground  LConnTagsString=a
  Conn1 : PMIOPort  Port=1  Side=Left
  Conn2 : PMIOPort  Port=2  Side=Left
  Conn3 : PMIOPort  Port=3  Side=Left
  wires:
  Current Measurement/1 -> Display1/1, Volts > pu1/1, Discrete  RMS value/1, Power/2(In2)
  Volts > pu1/1 -> Va (pu)1/1
  Va1/1 -> Display2/1, Power/1(In1), Discrete  RMS value1/1
  Discrete  RMS value/1 -> Va (pu)1/2
  Discrete  RMS value1/1 -> Va (pu)2/2, Volts > pu2/1
  Volts > pu2/1 -> Va (pu)2/1
  connections:
  Conn1/RConn1 -- Current Measurement/LConn1
  output Ground1/LConn1 -- Va1/LConn2
  Three-Phase Breaker2/RConn3 -- Three-Phase Series RLC Load- 0 -12/LConn3
  Three-Phase Breaker2/RConn2 -- Three-Phase Series RLC Load- 0 -12/LConn2
  Three-Phase Breaker2/RConn1 -- Three-Phase Series RLC Load- 0 -12/LConn1
  Three-Phase Breaker4/LConn3 -- Three-Phase Breaker1/LConn3 -- Three-Phase Breaker/LConn3 -- Va1/LConn1 -- Conn3/RConn1 -- Three-Phase Breaker2/LConn3
  Three-Phase Breaker2/LConn2 -- Conn2/RConn1 -- Three-Phase Breaker4/LConn2 -- Three-Phase Breaker1/LConn2 -- Three-Phase Breaker/LConn2
  Current Measurement/RConn1 -- Three-Phase Breaker2/LConn1 -- Three-Phase Breaker4/LConn1 -- Three-Phase Breaker1/LConn1 -- Three-Phase Breaker/LConn1
  Three-Phase Breaker4/RConn3 -- Three-Phase Series RLC Load- 9-12/LConn3
  Three-Phase Breaker4/RConn2 -- Three-Phase Series RLC Load- 9-12/LConn2
  Three-Phase Breaker4/RConn1 -- Three-Phase Series RLC Load- 9-12/LConn1
  Three-Phase Breaker1/RConn3 -- Three-Phase Series RLC Load- 6-9/LConn3
  Three-Phase Breaker1/RConn2 -- Three-Phase Series RLC Load- 6-9/LConn2
  Three-Phase Breaker1/RConn1 -- Three-Phase Series RLC Load- 6-9/LConn1
  Three-Phase Breaker/RConn3 -- Three-Phase Series RLC Load- 3-6/LConn3
  Three-Phase Breaker/RConn2 -- Three-Phase Series RLC Load- 3-6/LConn2
  Three-Phase Breaker/RConn1 -- Three-Phase Series RLC Load- 3-6/LConn1

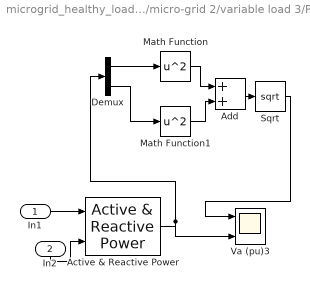
== system microgrid_healthy_load_profiling_with_Utility/micro-grid 2/variable load 3/Power ==
  In1 : Inport
  In2 : Inport  Port=2
  Active & Reactive Power : powerlib_extras/Measurements/Active & Reactive Power  f1=60
  Add : Sum
  Demux : Demux  Outputs=2
  Math Function : Math  Operator=square  OutputSignalType=real  SaturateOnIntegerOverflow=on
  Math Function1 : Math  Operator=square  OutputSignalType=real  SaturateOnIntegerOverflow=on
  Sqrt : Sqrt  SaturateOnIntegerOverflow=on
  Va (pu)3 : Scope  NumInputPorts=2
      settings: TickLabels=on  TimeRange=2  YMin=-175000~-5  YMax=225000~5  SaveName=vf3
  wires:
  Active & Reactive Power/1 -> Demux/1, Va (pu)3/2
  Demux/1 -> Math Function/1
  Math Function/1 -> Add/1
  Demux/2 -> Math Function1/1
  Math Function1/1 -> Add/2
  Add/1 -> Sqrt/1
  Sqrt/1 -> Va (pu)3/1
  In1/1 -> Active & Reactive Power/1
  In2/1 -> Active & Reactive Power/2

== system microgrid_healthy_load_profiling_with_Utility/micro-grid 2/variable load 4/Power ==
  In1 : Inport
  In2 : Inport  Port=2
  Active & Reactive Power : powerlib_extras/Measurements/Active & Reactive Power  f1=60
  Add : Sum
  Demux : Demux  Outputs=2
  Math Function : Math  Operator=square  OutputSignalType=real  SaturateOnIntegerOverflow=on
  Math Function1 : Math  Operator=square  OutputSignalType=real  SaturateOnIntegerOverflow=on
  Sqrt : Sqrt  SaturateOnIntegerOverflow=on
  Va (pu)3 : Scope  NumInputPorts=2
      settings: TickLabels=on  TimeRange=2  YMin=-175000~-5  YMax=225000~5  SaveName=vf3
  wires:
  Active & Reactive Power/1 -> Demux/1, Va (pu)3/2
  Demux/1 -> Math Function/1
  Math Function/1 -> Add/1
  Demux/2 -> Math Function1/1
  Math Function1/1 -> Add/2
  Add/1 -> Sqrt/1
  Sqrt/1 -> Va (pu)3/1
  In1/1 -> Active & Reactive Power/1
  In2/1 -> Active & Reactive Power/2

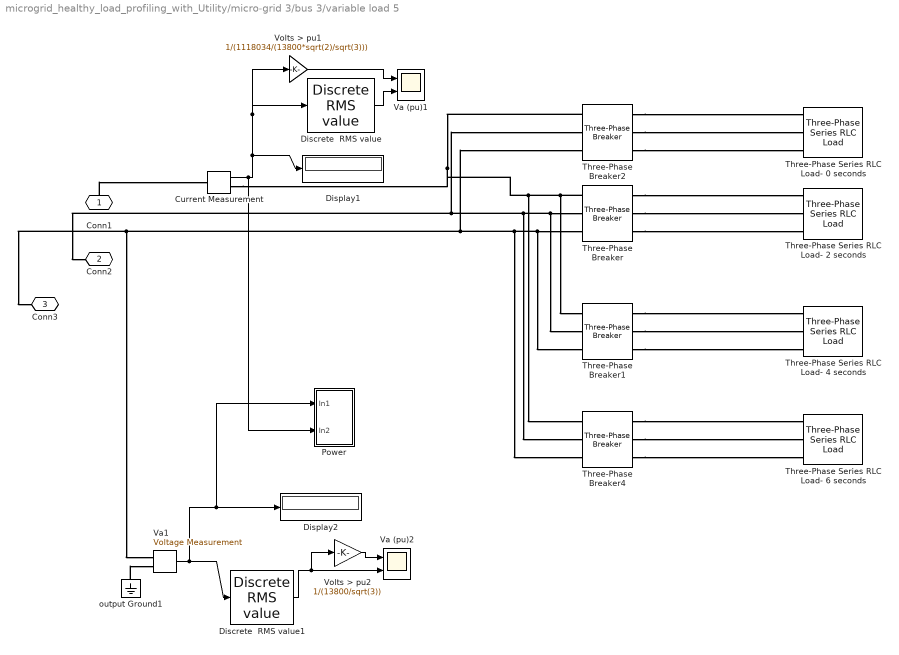
== system microgrid_healthy_load_profiling_with_Utility/micro-grid 3/bus 3/variable load 5 ==
  Current Measurement : powerlib/Measurements/Current Measurement  PhasorSimulation=off  OutputType=Complex  PSBequivalent=0
  Discrete  RMS value : powerlib_extras/Discrete Measurements/Discrete  RMS value  Freq=60  Mag_Init=0  Ts=Ts
  Discrete  RMS value1 : powerlib_extras/Discrete Measurements/Discrete  RMS value  Freq=60  Mag_Init=0  Ts=Ts
  Display1 : Display
  Display2 : Display
  Power : Subsystem
  Three-Phase Series RLC Load- 0 seconds : powerlib/Elements/Three-Phase Series RLC Load  LConnTagsString=A|B|C  Configuration=Y (grounded)  NominalVoltage=13800  NominalFrequency=60  ActivePower=150e3  InductivePower=10e3  CapacitivePower=0  Measurements=None  LoadType=constant Z
  "Three-Phase Series RLC Load- 2 seconds " : powerlib/Elements/Three-Phase Series RLC Load  LConnTagsString=A|B|C  Configuration=Y (grounded)  NominalVoltage=13800  NominalFrequency=60  ActivePower=50e3  InductivePower=0  CapacitivePower=0  Measurements=None  LoadType=constant Z
  Three-Phase Series RLC Load- 4 seconds : powerlib/Elements/Three-Phase Series RLC Load  LConnTagsString=A|B|C  Configuration=Y (grounded)  NominalVoltage=13800  NominalFrequency=60  ActivePower=100e3  InductivePower=1e3  CapacitivePower=0  Measurements=None  LoadType=constant Z
  Three-Phase Series RLC Load- 6 seconds : powerlib/Elements/Three-Phase Series RLC Load  LConnTagsString=A|B|C  Configuration=Y (grounded)  NominalVoltage=13800  NominalFrequency=60  ActivePower=75e3  InductivePower=10e3  CapacitivePower=0  Measurements=None  LoadType=constant Z
  Three-Phase Breaker : powerlib/Elements/Three-Phase Breaker  InitialState=open  SwitchA=on  SwitchB=on  SwitchC=on  SwitchTimes="[180/60  360/60]"  External=off  BreakerResistance=0.001  SnubberResistance=1e6  SnubberCapacitance=inf  Measurements=None
  Three-Phase Breaker1 : powerlib/Elements/Three-Phase Breaker  InitialState=open  SwitchA=on  SwitchB=on  SwitchC=on  SwitchTimes="[360/60  540/60]"  External=off  BreakerResistance=0.001  SnubberResistance=1e6  SnubberCapacitance=inf  Measurements=None
  Three-Phase Breaker2 : powerlib/Elements/Three-Phase Breaker  InitialState=closed  SwitchA=off  SwitchB=off  SwitchC=off  SwitchTimes=[120/60 ]  External=off  BreakerResistance=0.001  SnubberResistance=1e6  SnubberCapacitance=inf  Measurements=None
  Three-Phase Breaker4 : powerlib/Elements/Three-Phase Breaker  InitialState=open  SwitchA=on  SwitchB=on  SwitchC=on  SwitchTimes=[540/60]  External=off  BreakerResistance=0.001  SnubberResistance=1e6  SnubberCapacitance=inf  Measurements=None
  Va (pu)1 : Scope  NumInputPorts=2
      settings: TickLabels=on  TimeRange=2  YMin=-0.8~-50  YMax=0.8~50  SaveName=vf6
  Va (pu)2 : Scope  NumInputPorts=2
      settings: TickLabels=on  TimeRange=2  YMin=-2~-12500  YMax=2~12500  SaveName=vf2
  Va1 : powerlib/Measurements/Voltage Measurement  Tag=PoWeRsYsTeMmEaSuReMeNt  PhasorSimulation=off  OutputType=Magnitude  PSBequivalent=0
  Volts > pu1 : Gain  Gain=1/(1118034/(13800*sqrt(2)/sqrt(3)))  SaturateOnIntegerOverflow=on  OutDataTypeStr=Inherit: Same as input  ParamDataTypeStr=Inherit: Same as input
  Volts > pu2 : Gain  Gain=1/(13800/sqrt(3))  SaturateOnIntegerOverflow=on  OutDataTypeStr=Inherit: Same as input  ParamDataTypeStr=Inherit: Same as input
  output Ground1 : powerlib/Elements/Ground  LConnTagsString=a
  Conn1 : PMIOPort  Port=1  Side=Left
  Conn2 : PMIOPort  Port=2  Side=Left
  Conn3 : PMIOPort  Port=3  Side=Left
  wires:
  Va1/1 -> Display2/1, Power/1(In1), Discrete  RMS value1/1
  Volts > pu1/1 -> Va (pu)1/1
  Current Measurement/1 -> Volts > pu1/1, Discrete  RMS value/1, Display1/1, Power/2(In2)
  Discrete  RMS value/1 -> Va (pu)1/2
  Discrete  RMS value1/1 -> Va (pu)2/2, Volts > pu2/1
  Volts > pu2/1 -> Va (pu)2/1
  connections:
  Three-Phase Breaker/RConn1 -- "Three-Phase Series RLC Load- 2 seconds "/LConn1
  Three-Phase Breaker/RConn2 -- "Three-Phase Series RLC Load- 2 seconds "/LConn2
  Three-Phase Breaker/RConn3 -- "Three-Phase Series RLC Load- 2 seconds "/LConn3
  Three-Phase Breaker1/RConn1 -- Three-Phase Series RLC Load- 4 seconds/LConn1
  Three-Phase Breaker1/RConn2 -- Three-Phase Series RLC Load- 4 seconds/LConn2
  Three-Phase Breaker1/RConn3 -- Three-Phase Series RLC Load- 4 seconds/LConn3
  Three-Phase Breaker4/RConn1 -- Three-Phase Series RLC Load- 6 seconds/LConn1
  Three-Phase Breaker4/RConn2 -- Three-Phase Series RLC Load- 6 seconds/LConn2
  Three-Phase Breaker4/RConn3 -- Three-Phase Series RLC Load- 6 seconds/LConn3
  Three-Phase Breaker/LConn1 -- Three-Phase Breaker1/LConn1 -- Three-Phase Breaker4/LConn1 -- Three-Phase Breaker2/LConn1 -- Current Measurement/RConn1
  Three-Phase Breaker/LConn2 -- Three-Phase Breaker1/LConn2 -- Three-Phase Breaker4/LConn2 -- Conn2/RConn1 -- Three-Phase Breaker2/LConn2
  Three-Phase Breaker/LConn3 -- Three-Phase Breaker1/LConn3 -- Three-Phase Breaker4/LConn3 -- Three-Phase Breaker2/LConn3 -- Conn3/RConn1 -- Va1/LConn1
  Three-Phase Breaker2/RConn1 -- Three-Phase Series RLC Load- 0 seconds/LConn1
  Three-Phase Breaker2/RConn2 -- Three-Phase Series RLC Load- 0 seconds/LConn2
  Three-Phase Breaker2/RConn3 -- Three-Phase Series RLC Load- 0 seconds/LConn3
  output Ground1/LConn1 -- Va1/LConn2
  Conn1/RConn1 -- Current Measurement/LConn1
